simulink model "Attitude_control_RW"  (R2021b)
settings: Solver=VariableStepAuto  StartTime=0.0  StopTime=20  FixedStep=0.0001  RelTol=1e-3
values from neighbouring files (symbols this model uses):
  D = 9.4e-5*Kt    (= 4.7e-06)    [motor_parameter.m]
  J = 1.94e-4*Kt    (= 9.7e-06)    [motor_parameter.m]
  kii = (J*(-Kt^2+kpo*R)*wn^2)/(Kt*(D^2+kpo^2+J^2*wn^2-2*J*kpo*wn*zeta+2*D*(kpo-J*wn*zeta)))    (= 0.394297267374)    [motor_parameter.m]
  kpi = -(D^2*R+J^2*R*wn^2+kpo*(Kt^2-2*J*R*wn*zeta)+D*(Kt^2+R*(kpo-2*J*wn*zeta))/(Kt*(D^2+kpo^2+J^2*wn^2-2*J*kpo*wn*zeta+2*D*(kpo-J*wn*zeta))))    (= 0.0794485412984)    [motor_parameter.m]
  kpo = 10    [motor_parameter.m]
  Kt = 0.05    [motor_parameter.m]
  L = 0.001    [motor_parameter.m]
  R = 14.3    [motor_parameter.m]
  Tc = 0.053*Kt    (= 0.00265)    [motor_parameter.m]
undefined symbols (not defined in the file or in its folder): b, Is, kk, Km, Q, q_init, Rgyro, Rstr, rw_Inertia, rw_SensorToBody, Ts, unit7, w0, w_dot_init, w_init, wRW_init
libraries: simulink_extras x13, sharedtransform x12, simulink x4, slpidlib x3, aerolibutil x2, sharedTrackingLibrary x1
(part 2 of 2)

== system Attitude_control_RW/Dynamic/Subsystem ==
  qest : Inport
  Quaternions to Direction Cosine Matrix : sharedtransform/Quaternions to  Direction Cosine Matrix  aMode=aMode
      settings: SourceProductBaseCode=AE,PW,DR,MT,UV,VE
  Subsystem : Subsystem
  "DCM " : Outport  VectorParamsAs1DForOutWhenUnconnected=off
  wires:
  Quaternions to Direction Cosine Matrix/1 -> "DCM "/1
  Subsystem/1(q0,q1,q2,q3) -> Quaternions to Direction Cosine Matrix/1
  qest/1 -> Subsystem/1(q1,q2,q3,q4)

== system Attitude_control_RW/Dynamic/Subsystem1 ==
  "DCM " : Inport
  Direction Cosine Matrix to Rotation Angles : sharedtransform/Direction Cosine Matrix to Rotation Angles  rotationOrder=ZYX  aMode=aMode  action=None  tolerance=eps(2)
      settings: SourceProductBaseCode=AE,PW,DR,MT,UV,VE
  Radians to Degrees1 : simulink_extras/Transformations/Radians to Degrees
  Euler Angle : Outport  VectorParamsAs1DForOutWhenUnconnected=off
  wires:
  Radians to Degrees1/1 -> Euler Angle/1
  Direction Cosine Matrix to Rotation Angles/1 -> Radians to Degrees1/1
  "DCM "/1 -> Direction Cosine Matrix to Rotation Angles/1

== system Attitude_control_RW/Satellite Kinematic & Dynamic Model/Dynamic Model ==
  Mc+Md : Inport
  "Hrw_B " : Inport  Port=2
  Add : Sum  Inputs=-+
  Add1 : Sum
  Embedded MATLAB Function : MATLAB Function  TreatAsAtomicUnit=on
  IC : InitialCondition  Value=w_init
  IC1 : InitialCondition  Value=w_dot_init
  Inertia Matrix : Constant  Value=Is  VectorParams1D=off
  Integrator : Integrator  InitialConditionSource=external  InitialCondition=[0;0;0]
  Invert 3x3 Matrix : aerolibutil/Invert  3x3 Matrix
  Product : Product  Multiplication=Matrix(*)  RndMeth=Zero
  Product1 : Product  Multiplication=Matrix(*)  RndMeth=Zero
  Reshape : Reshape  OutputDimensionality=Column vector (2-D)
  Reshape1 : Reshape  OutputDimensionality=Column vector (2-D)
  w_initial : Constant  Value=w_init  VectorParams1D=off  SampleTime=-1
  w_IB_B : Outport  VectorParamsAs1DForOutWhenUnconnected=off
  wires:
  Inertia Matrix/1 -> Invert 3x3 Matrix/1, Product/1
  IC/1 -> Product/2, Embedded MATLAB Function/1(w)
  Mc+Md/1 -> Reshape1/1
  Invert 3x3 Matrix/1 -> Product1/1
  Integrator/1 -> w_IB_B/1, IC/1
  Product1/1 -> IC1/1
  Embedded MATLAB Function/1(y) -> Reshape/1
  w_initial/1 -> Integrator/2
  Add/1 -> Product1/2
  IC1/1 -> Integrator/1
  Reshape/1 -> Add/1
  Reshape1/1 -> Add/2
  Product/1 -> Add1/1
  Add1/1 -> Embedded MATLAB Function/2(Iw_plus_hwheel)
  "Hrw_B "/1 -> Add1/2

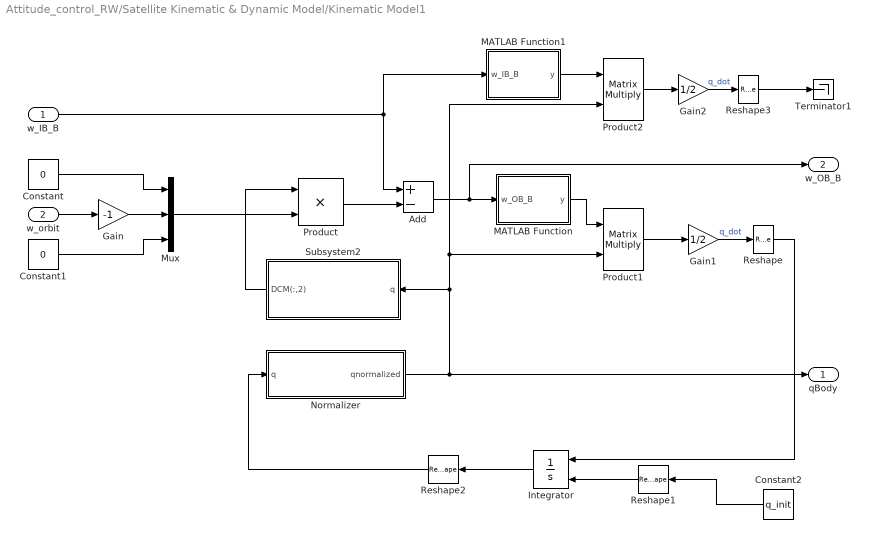
== system Attitude_control_RW/Satellite Kinematic & Dynamic Model/Kinematic Model1 ==
  w_IB_B : Inport
  w_orbit : Inport  Port=2
  Add : Sum  Inputs=+-
  Constant : Constant  Value=0
  Constant1 : Constant  Value=0
  Constant2 : Constant  Value=q_init
  Gain : Gain  Gain=-1
  Gain1 : Gain  Gain=1/2
  Gain2 : Gain  Gain=1/2
  Integrator : Integrator  InitialConditionSource=external
  MATLAB Function : MATLAB Function  TreatAsAtomicUnit=on
  MATLAB Function1 : MATLAB Function  TreatAsAtomicUnit=on
  Mux : Mux  Inputs=3
  Normalizer : MATLAB Function  TreatAsAtomicUnit=on
  Product : Product
  Product1 : Product  Multiplication=Matrix(*)
  Product2 : Product  Multiplication=Matrix(*)
  Reshape{,1..3} (4 alike) : Reshape  OutputDimensionality=Column vector (2-D)
  Subsystem2 : Subsystem
  Terminator1 : Terminator
  qBody : Outport  VectorParamsAs1DForOutWhenUnconnected=off
  w_OB_B : Outport  Port=2  VectorParamsAs1DForOutWhenUnconnected=off
  wires:
  Reshape2/1 -> Normalizer/1(q)
  Product/1 -> Add/2
  Integrator/1 -> Reshape2/1
  Normalizer/1(qnormalized) -> qBody/1, Subsystem2/1(q), Product1/2, Product2/2
  Reshape1/1 -> Integrator/2
  Add/1 -> MATLAB Function/1(w_OB_B), w_OB_B/1
  w_orbit/1 -> Gain/1
  Mux/1 -> Product/2
  Constant/1 -> Mux/1
  Constant1/1 -> Mux/3
  Product1/1 -> Gain1/1
  MATLAB Function/1(y) -> Product1/1
  Gain1/1 -> Reshape/1  "q_dot"
  w_IB_B/1 -> MATLAB Function1/1(w_IB_B), Add/1
  Product2/1 -> Gain2/1
  MATLAB Function1/1(y) -> Product2/1
  Gain2/1 -> Reshape3/1  "q_dot"
  Subsystem2/1(DCM(:,2)) -> Product/1
  Gain/1 -> Mux/2
  Reshape/1 -> Integrator/1
  Reshape3/1 -> Terminator1/1
  Constant2/1 -> Reshape1/1

== system Attitude_control_RW/Satellite Kinematic & Dynamic Model/Subsystem ==
  qest : Inport
  Quaternions to Direction Cosine Matrix : sharedtransform/Quaternions to  Direction Cosine Matrix  aMode=aMode
      settings: SourceProductBaseCode=AE
  Subsystem : Subsystem
  "DCM " : Outport  VectorParamsAs1DForOutWhenUnconnected=off
  wires:
  Quaternions to Direction Cosine Matrix/1 -> "DCM "/1
  Subsystem/1(q0,q1,q2,q3) -> Quaternions to Direction Cosine Matrix/1
  qest/1 -> Subsystem/1(q1,q2,q3,q4)

== system Attitude_control_RW/Satellite Kinematic & Dynamic Model/Subsystem1 ==
  "DCM " : Inport
  Direction Cosine Matrix to Rotation Angles : sharedtransform/Direction Cosine Matrix to Rotation Angles  rotationOrder=ZYX  aMode=aMode  action=None  tolerance=eps(2)
      settings: SourceProductBaseCode=AE
  Radians to Degrees1 : simulink_extras/Transformations/Radians to Degrees
  Euler Angle : Outport  VectorParamsAs1DForOutWhenUnconnected=off
  wires:
  Radians to Degrees1/1 -> Euler Angle/1
  Direction Cosine Matrix to Rotation Angles/1 -> Radians to Degrees1/1
  "DCM "/1 -> Direction Cosine Matrix to Rotation Angles/1

== system Attitude_control_RW/Sensor Measurement Model (GYRO + STR)/GYRO Sensor Model ==
  w_Body : Inport
  Gyroscope Model : Subsystem
  Zero-Order Hold2 : ZeroOrderHold  SampleTime=Ts
  w_Body_meas : Outport  VectorParamsAs1DForOutWhenUnconnected=off
  wires:
  w_Body/1 -> Gyroscope Model/1(w_Body)
  Gyroscope Model/1(Gyro1_wmeas) -> Zero-Order Hold2/1
  Zero-Order Hold2/1 -> w_Body_meas/1

== system Attitude_control_RW/Sensor Measurement Model (GYRO + STR)/Normalization Model ==
  u : Inport
  Divide : Product  Inputs=*/
  MATLAB Function : MATLAB Function  TreatAsAtomicUnit=on
  Math Function2 : Math  Operator=square  SignedPower=on  SaturateOnIntegerOverflow=on
  Sum of Elements : Sum  Inputs=+
  Normalized_u : Outport  VectorParamsAs1DForOutWhenUnconnected=off
  wires:
  Divide/1 -> Normalized_u/1
  MATLAB Function/1(y) -> Divide/2
  Sum of Elements/1 -> MATLAB Function/1(u)
  u/1 -> Divide/1, Math Function2/1
  Math Function2/1 -> Sum of Elements/1

== system Attitude_control_RW/Sensor Measurement Model (GYRO + STR)/Star Tracker Model ==
  q_Body : Inport
  Scope : Scope
  StarTracker 1 Error Model3 : Subsystem  TreatAsAtomicUnit=on
  Zero-Order Hold2 : ZeroOrderHold  SampleTime=0.1
  q_Body_meas : Outport  VectorParamsAs1DForOutWhenUnconnected=off
  wires:
  Zero-Order Hold2/1 -> Scope/1, q_Body_meas/1
  q_Body/1 -> StarTracker 1 Error Model3/1("q_Body ")
  StarTracker 1 Error Model3/1("q_body_meas ") -> Zero-Order Hold2/1

== system Attitude_control_RW/Subsystem/Subsystem1 ==
  q0,q1,q2,q3 : Inport
  Demux1 : Demux
  Mux1 : Mux
  q1,q2,q3,q4 : Outport  VectorParamsAs1DForOutWhenUnconnected=off
  wires:
  q0,q1,q2,q3/1 -> Demux1/1
  Mux1/1 -> q1,q2,q3,q4/1
  Demux1/1 -> Mux1/4
  Demux1/2 -> Mux1/1
  Demux1/3 -> Mux1/2
  Demux1/4 -> Mux1/3

== system Attitude_control_RW/Subsystem1/Subsystem1 ==
  q0,q1,q2,q3 : Inport
  Demux1 : Demux
  Mux1 : Mux
  q1,q2,q3,q4 : Outport  VectorParamsAs1DForOutWhenUnconnected=off
  wires:
  q0,q1,q2,q3/1 -> Demux1/1
  Mux1/1 -> q1,q2,q3,q4/1
  Demux1/1 -> Mux1/4
  Demux1/2 -> Mux1/1
  Demux1/3 -> Mux1/2
  Demux1/4 -> Mux1/3

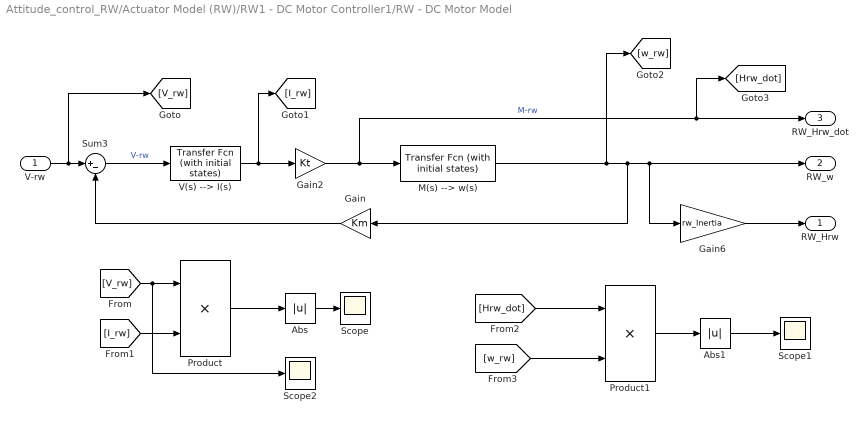
== system Attitude_control_RW/Actuator Model (RW)/RW1 - DC Motor Controller1/RW - DC Motor Model ==
  V-rw : Inport
  Abs : Abs
  Abs1 : Abs
  Gain : Gain  Gain=Km
  Gain2 : Gain  Gain=Kt
  Gain6 : Gain  Gain=rw_Inertia
  M(s) --> w(s) : simulink_extras/Additional Linear/Transfer Fcn (with initial states)  N=[1]  D=[5e-4 b]  X0=0
  Product : Product
  Product1 : Product
  Scope : Scope
  Scope1 : Scope
  Scope2 : Scope
  Sum3 : Sum  Inputs=|+-
  V(s) --> I(s) : simulink_extras/Additional Linear/Transfer Fcn (with initial states)  N=1  D=[R]  X0=0
  RW_Hrw : Outport  VectorParamsAs1DForOutWhenUnconnected=off
  RW_w : Outport  Port=2  VectorParamsAs1DForOutWhenUnconnected=off
  RW_Hrw_dot : Outport  Port=3  VectorParamsAs1DForOutWhenUnconnected=off
  wires:
  V-rw/1 -> [V_rw], Sum3/1
  Gain2/1 -> M(s) --> w(s)/1, [Hrw_dot], RW_Hrw_dot/1  "M-rw"
  Gain6/1 -> RW_Hrw/1
  Gain/1 -> Sum3/2
  Sum3/1 -> V(s) --> I(s)/1  "V-rw"
  V(s) --> I(s)/1 -> [I_rw], Gain2/1
  M(s) --> w(s)/1 -> RW_w/1, Gain6/1, Gain/1, [w_rw]
  [V_rw] -> Scope2/1, Product/1
  [I_rw] -> Product/2
  Product/1 -> Abs/1
  Abs/1 -> Scope/1
  [Hrw_dot] -> Product1/1
  [w_rw] -> Product1/2
  Product1/1 -> Abs1/1
  Abs1/1 -> Scope1/1

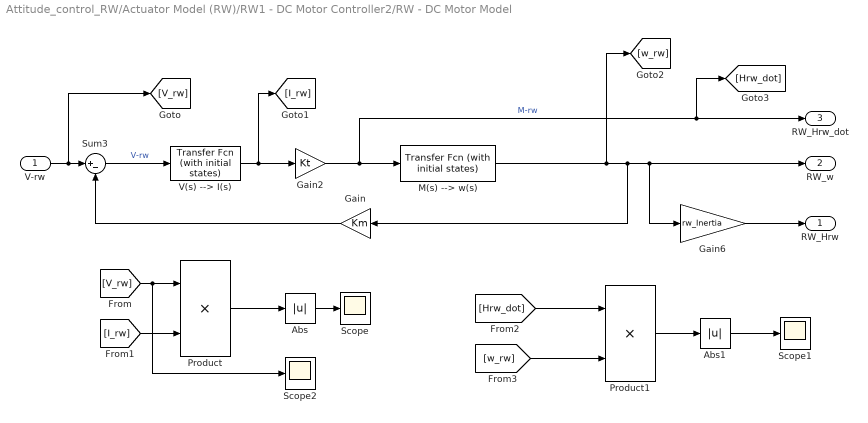
== system Attitude_control_RW/Actuator Model (RW)/RW1 - DC Motor Controller2/RW - DC Motor Model ==
  V-rw : Inport
  Abs : Abs
  Abs1 : Abs
  Gain : Gain  Gain=Km
  Gain2 : Gain  Gain=Kt
  Gain6 : Gain  Gain=rw_Inertia
  M(s) --> w(s) : simulink_extras/Additional Linear/Transfer Fcn (with initial states)  N=[1]  D=[5e-4 b]  X0=0
  Product : Product
  Product1 : Product
  Scope : Scope
  Scope1 : Scope
  Scope2 : Scope
  Sum3 : Sum  Inputs=|+-
  V(s) --> I(s) : simulink_extras/Additional Linear/Transfer Fcn (with initial states)  N=1  D=[R]  X0=0
  RW_Hrw : Outport  VectorParamsAs1DForOutWhenUnconnected=off
  RW_w : Outport  Port=2  VectorParamsAs1DForOutWhenUnconnected=off
  RW_Hrw_dot : Outport  Port=3  VectorParamsAs1DForOutWhenUnconnected=off
  wires:
  V-rw/1 -> [V_rw], Sum3/1
  Gain2/1 -> M(s) --> w(s)/1, [Hrw_dot], RW_Hrw_dot/1  "M-rw"
  Gain6/1 -> RW_Hrw/1
  Gain/1 -> Sum3/2
  Sum3/1 -> V(s) --> I(s)/1  "V-rw"
  V(s) --> I(s)/1 -> [I_rw], Gain2/1
  M(s) --> w(s)/1 -> RW_w/1, Gain6/1, Gain/1, [w_rw]
  [V_rw] -> Scope2/1, Product/1
  [I_rw] -> Product/2
  Product/1 -> Abs/1
  Abs/1 -> Scope/1
  [Hrw_dot] -> Product1/1
  [w_rw] -> Product1/2
  Product1/1 -> Abs1/1
  Abs1/1 -> Scope1/1

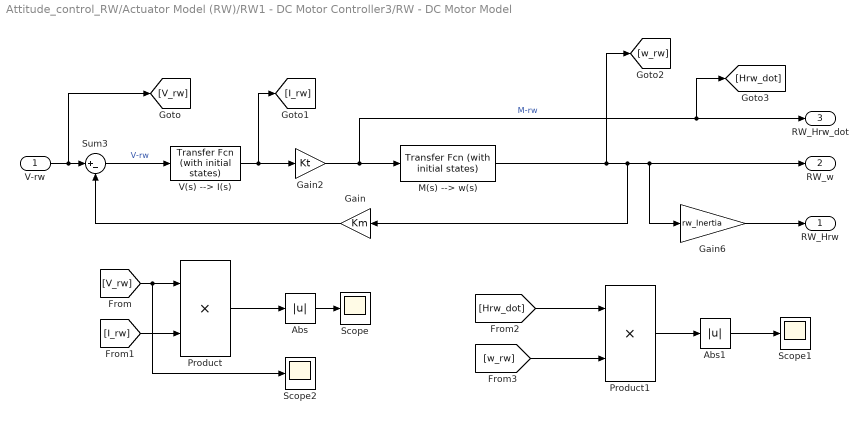
== system Attitude_control_RW/Actuator Model (RW)/RW1 - DC Motor Controller3/RW - DC Motor Model ==
  V-rw : Inport
  Abs : Abs
  Abs1 : Abs
  Gain : Gain  Gain=Km
  Gain2 : Gain  Gain=Kt
  Gain6 : Gain  Gain=rw_Inertia
  M(s) --> w(s) : simulink_extras/Additional Linear/Transfer Fcn (with initial states)  N=[1]  D=[5e-4 b]  X0=0
  Product : Product
  Product1 : Product
  Scope : Scope
  Scope1 : Scope
  Scope2 : Scope
  Sum3 : Sum  Inputs=|+-
  V(s) --> I(s) : simulink_extras/Additional Linear/Transfer Fcn (with initial states)  N=1  D=[R]  X0=0
  RW_Hrw : Outport  VectorParamsAs1DForOutWhenUnconnected=off
  RW_w : Outport  Port=2  VectorParamsAs1DForOutWhenUnconnected=off
  RW_Hrw_dot : Outport  Port=3  VectorParamsAs1DForOutWhenUnconnected=off
  wires:
  V-rw/1 -> [V_rw], Sum3/1
  Gain2/1 -> M(s) --> w(s)/1, [Hrw_dot], RW_Hrw_dot/1  "M-rw"
  Gain6/1 -> RW_Hrw/1
  Gain/1 -> Sum3/2
  Sum3/1 -> V(s) --> I(s)/1  "V-rw"
  V(s) --> I(s)/1 -> [I_rw], Gain2/1
  M(s) --> w(s)/1 -> RW_w/1, Gain6/1, Gain/1, [w_rw]
  [V_rw] -> Scope2/1, Product/1
  [I_rw] -> Product/2
  Product/1 -> Abs/1
  Abs/1 -> Scope/1
  [Hrw_dot] -> Product1/1
  [w_rw] -> Product1/2
  Product1/1 -> Abs1/1
  Abs1/1 -> Scope1/1

== system Attitude_control_RW/Actuator Model (RW)/RW1 - DC Motor Controller5/RW - DC Motor Model ==
  V-rw : Inport
  Abs : Abs
  Abs1 : Abs
  Gain : Gain  Gain=Km
  Gain2 : Gain  Gain=Kt
  Gain6 : Gain  Gain=rw_Inertia
  M(s) --> w(s) : simulink_extras/Additional Linear/Transfer Fcn (with initial states)  N=[1]  D=[5e-4 b]  X0=0
  Product : Product
  Product1 : Product
  Scope : Scope
  Scope1 : Scope
  Scope2 : Scope
  Sum3 : Sum  Inputs=|+-
  V(s) --> I(s) : simulink_extras/Additional Linear/Transfer Fcn (with initial states)  N=1  D=[R]  X0=0
  RW_Hrw : Outport  VectorParamsAs1DForOutWhenUnconnected=off
  RW_w : Outport  Port=2  VectorParamsAs1DForOutWhenUnconnected=off
  RW_Hrw_dot : Outport  Port=3  VectorParamsAs1DForOutWhenUnconnected=off
  wires:
  V-rw/1 -> [V_rw], Sum3/1
  Gain2/1 -> M(s) --> w(s)/1, [Hrw_dot], RW_Hrw_dot/1  "M-rw"
  Gain6/1 -> RW_Hrw/1
  Gain/1 -> Sum3/2
  Sum3/1 -> V(s) --> I(s)/1  "V-rw"
  V(s) --> I(s)/1 -> [I_rw], Gain2/1
  M(s) --> w(s)/1 -> RW_w/1, Gain6/1, Gain/1, [w_rw]
  [V_rw] -> Scope2/1, Product/1
  [I_rw] -> Product/2
  Product/1 -> Abs/1
  Abs/1 -> Scope/1
  [Hrw_dot] -> Product1/1
  [w_rw] -> Product1/2
  Product1/1 -> Abs1/1
  Abs1/1 -> Scope1/1

== system Attitude_control_RW/Controller/Subsystem/Subsystem1 ==
  q0,q1,q2,q3 : Inport
  Demux1 : Demux
  Mux1 : Mux
  q1,q2,q3,q4 : Outport  VectorParamsAs1DForOutWhenUnconnected=off
  wires:
  q0,q1,q2,q3/1 -> Demux1/1
  Mux1/1 -> q1,q2,q3,q4/1
  Demux1/1 -> Mux1/4
  Demux1/2 -> Mux1/1
  Demux1/3 -> Mux1/2
  Demux1/4 -> Mux1/3

== system Attitude_control_RW/Dynamic/Kinematic Model1/Subsystem2 ==
  q : Inport
  MATLAB Function : MATLAB Function  TreatAsAtomicUnit=on
  Quaternions to Direction Cosine Matrix : sharedtransform/Quaternions to  Direction Cosine Matrix  aMode=aMode
      settings: SourceProductBaseCode=AE,PW,DR,MT,UV,VE
  Reshape2 : Reshape  OutputDimensionality=Column vector (2-D)
  Subsystem : Subsystem
  DCM(:,2) : Outport  VectorParamsAs1DForOutWhenUnconnected=off
  wires:
  Subsystem/1(q0,q1,q2,q3) -> Quaternions to Direction Cosine Matrix/1
  q/1 -> Subsystem/1(q1,q2,q3,q4)
  Quaternions to Direction Cosine Matrix/1 -> MATLAB Function/1(DCM)
  MATLAB Function/1(DCM_2) -> Reshape2/1
  Reshape2/1 -> DCM(:,2)/1

== system Attitude_control_RW/Dynamic/Subsystem/Subsystem ==
  q1,q2,q3,q4 : Inport
  Demux1 : Demux
  Mux1 : Mux
  q0,q1,q2,q3 : Outport  VectorParamsAs1DForOutWhenUnconnected=off
  wires:
  Demux1/2 -> Mux1/3
  q1,q2,q3,q4/1 -> Demux1/1
  Mux1/1 -> q0,q1,q2,q3/1
  Demux1/4 -> Mux1/1
  Demux1/1 -> Mux1/2
  Demux1/3 -> Mux1/4

== system Attitude_control_RW/Satellite Kinematic & Dynamic Model/Kinematic Model1/Subsystem2 ==
  q : Inport
  MATLAB Function : MATLAB Function  TreatAsAtomicUnit=on
  Quaternions to Direction Cosine Matrix : sharedtransform/Quaternions to  Direction Cosine Matrix  aMode=aMode
      settings: SourceProductBaseCode=AE
  Reshape2 : Reshape  OutputDimensionality=Column vector (2-D)
  Subsystem : Subsystem
  DCM(:,2) : Outport  VectorParamsAs1DForOutWhenUnconnected=off
  wires:
  Subsystem/1(q0,q1,q2,q3) -> Quaternions to Direction Cosine Matrix/1
  q/1 -> Subsystem/1(q1,q2,q3,q4)
  Quaternions to Direction Cosine Matrix/1 -> MATLAB Function/1(DCM)
  MATLAB Function/1(DCM_2) -> Reshape2/1
  Reshape2/1 -> DCM(:,2)/1

== system Attitude_control_RW/Satellite Kinematic & Dynamic Model/Subsystem/Subsystem ==
  q1,q2,q3,q4 : Inport
  Demux1 : Demux
  Mux1 : Mux
  q0,q1,q2,q3 : Outport  VectorParamsAs1DForOutWhenUnconnected=off
  wires:
  Demux1/2 -> Mux1/3
  q1,q2,q3,q4/1 -> Demux1/1
  Mux1/1 -> q0,q1,q2,q3/1
  Demux1/4 -> Mux1/1
  Demux1/1 -> Mux1/2
  Demux1/3 -> Mux1/4

== system Attitude_control_RW/Sensor Measurement Model (GYRO + STR)/GYRO Sensor Model/Gyroscope Model ==
  w_Body : Inport
  Add : Sum
  Band-Limited White Noise : simulink/Sources/Band-Limited White Noise  Cov=Rgyro*Ts  Ts=Ts  seed=[23341]
  Saturation1 : Saturate  UpperLimit=abs(1000)  LowerLimit=-abs(1000)
  Gyro1_wmeas : Outport  VectorParamsAs1DForOutWhenUnconnected=off
  wires:
  Add/1 -> Saturation1/1
  Saturation1/1 -> Gyro1_wmeas/1
  w_Body/1 -> Add/1
  Band-Limited White Noise/1 -> Add/2

== system Attitude_control_RW/Sensor Measurement Model (GYRO + STR)/Star Tracker Model/StarTracker 1 Error Model3 ==
  "q_Body " : Inport
  Add : Sum
  Band-Limited White Noise : simulink/Sources/Band-Limited White Noise  Cov=Rstr*Ts  Ts=Ts  seed=[12345]
  "q_body_meas " : Outport  VectorParamsAs1DForOutWhenUnconnected=off
  wires:
  Band-Limited White Noise/1 -> Add/2
  "q_Body "/1 -> Add/1
  Add/1 -> "q_body_meas "/1

== system Attitude_control_RW/Dynamic/Kinematic Model1/Subsystem2/Subsystem ==
  q1,q2,q3,q4 : Inport
  Demux1 : Demux
  Mux1 : Mux
  q0,q1,q2,q3 : Outport  VectorParamsAs1DForOutWhenUnconnected=off
  wires:
  Demux1/2 -> Mux1/3
  q1,q2,q3,q4/1 -> Demux1/1
  Mux1/1 -> q0,q1,q2,q3/1
  Demux1/4 -> Mux1/1
  Demux1/1 -> Mux1/2
  Demux1/3 -> Mux1/4

== system Attitude_control_RW/Satellite Kinematic & Dynamic Model/Kinematic Model1/Subsystem2/Subsystem ==
  q1,q2,q3,q4 : Inport
  Demux1 : Demux
  Mux1 : Mux
  q0,q1,q2,q3 : Outport  VectorParamsAs1DForOutWhenUnconnected=off
  wires:
  Demux1/2 -> Mux1/3
  q1,q2,q3,q4/1 -> Demux1/1
  Mux1/1 -> q0,q1,q2,q3/1
  Demux1/4 -> Mux1/1
  Demux1/1 -> Mux1/2
  Demux1/3 -> Mux1/4

== matlab function Attitude_control_RW/Satellite Kinematic & Dynamic Model/Kinematic Model1/Normalizer ==
  data: qnormalized output; q input
function qnormalized = fcn(q)

%Normalizes the quaternion

qnormalized = q;
qs = q(4);
qv = [q(1); q(2); q(3)];

qnormalized(4)= qs /norm(q);
qnormalized(1)= qv(1)/norm(q);
qnormalized(2)= qv(2)/norm(q);
qnormalized(3)= qv(3)/norm(q);

== matlab function Attitude_control_RW/Dynamic/Kinematic Model1/MATLAB Function1 ==
  data: w_IB_B input; y output
function y = skew_wIB_B(w_IB_B)


y = [0, w_IB_B(3,1), -w_IB_B(2,1), w_IB_B(1,1);...
    -w_IB_B(3,1), 0, w_IB_B(1,1), w_IB_B(2,1);...
     w_IB_B(2,1), -w_IB_B(1,1), 0, w_IB_B(3,1);...
    -w_IB_B(1,1), -w_IB_B(2,1), -w_IB_B(3,1), 0];
end

== matlab function Attitude_control_RW/Actuator Model (RW)/Reaction Wheel Model ==
  data: rw_SensorToBody input; Hrw_dot_des output; inv_rwSensorToBody input; Mc input; w_IB_B input; wRw input
function Hrw_dot_des = rwModel(rw_SensorToBody,inv_rwSensorToBody,Mc,w_IB_B,wRw)
% The desired torque is calculated for each reaction wheel 

% The required momentum input
% wRw               (4x1) matrix
% rwInertia_matrix  (4x4) matrix
% rw_SensorToBody   (3x4) matrix
rwInertia = 5e-4; % RW moment of inertia (kg-m2)
rwInertia_matrix = eye(4,4)* rwInertia;
Hrw = rwInertia_matrix * wRw; 

% Hrw_B     (3x1) matrix
% Hrw_B_dot (3x1) matrix
% From Actuator Frame to Satellite Body Frame
Hrw_B = rw_SensorToBody * Hrw ;

% Desired reaction wheel torque in Body Frame
Hrw_B_dot = Mc + cross(w_IB_B,Hrw_B) ;

% Desired reaction wheel torque in Actuator Frame
Hrw_dot_des = inv_rwSensorToBody * Hrw_B_dot ; 

end

== matlab function Attitude_control_RW/Actuator Model (RW)/RW1 - DC Motor Controller5/MATLAB Function1 ==
  data: y output
function y = fcn()
sigma = 2;
y = sigma*randn;

== matlab function Attitude_control_RW/MATLAB Function ==
  data: qref input; qerr_xyz output; qest input
function qerr_xyz  = quaternionError(qref, qest)

qerr = [qest(4)  qest(3) -qest(2) qest(1);...
       -qest(3)  qest(4)  qest(1) qest(2);...
        qest(2) -qest(1)  qest(4) qest(3);...
       -qest(1) -qest(2) -qest(3) qest(4)]*[-qref(1);-qref(2);-qref(3);qref(4)]; % Verify

qerr_xyz = [qerr(1,1); qerr(2,1); qerr(3,1)];     
% qerr_x = qerr(1,1);
% qerr_y = qerr(2,1);
% qerr_z = qerr(3,1);
qerr_4 = qerr(4,1);
qerr_xyz*qerr_4;

end
% % 
% function qerr_xyz  = quaternionError(qref, qest)
% 
% qerr = [qref(4)  -qref(3) qref(2) qref(1);...
%         qref(3)  qref(4)  -qref(1) qref(2);...
%         -qref(2) qref(1)  qref(4) qref(3);...
%        -qref(1) -qref(2) -qref(3) qref(4)]*[-qest(1);-qest(2);-qest(3);qest(4)];
% 
% qerr_xyz = [qerr(1,1); qerr(2,1); qerr(3,1)];     
% % qerr_x = qerr(1,1);
% % qerr_y = qerr(2,1);
% % qerr_z = qerr(3,1);
% 
% end

== matlab function Attitude_control_RW/Sensor Measurement Model (GYRO + STR)/Normalization Model/MATLAB Function ==
  data: u input; y output
function y = Sqrt(u)
%#codegen

y = sqrt(u);

== matlab function Attitude_control_RW/Actuator Model (RW)/RW1 - DC Motor Controller5/MATLAB Function ==
  data: y output
function y = fcn()
sigma = 0.1;
y = sigma*randn;

== matlab function Attitude_control_RW/Controller/MATLAB Function ==
  data: qref input; qerr_xyz output; qest input
function qerr_xyz  = quaternionError(qref, qest)

qerr = [qest(4)  qest(3) -qest(2) qest(1);...
       -qest(3)  qest(4)  qest(1) qest(2);...
        qest(2) -qest(1)  qest(4) qest(3);...
       -qest(1) -qest(2) -qest(3) qest(4)]*[-qref(1);-qref(2);-qref(3);qref(4)]; % Verify

qerr_xyz = [qerr(1,1); qerr(2,1); qerr(3,1)];     
% qerr_x = qerr(1,1);
% qerr_y = qerr(2,1);
% qerr_z = qerr(3,1);
qerr_4 = qerr(4,1);
qerr_xyz*qerr_4;

end
% % 
% function qerr_xyz  = quaternionError(qref, qest)
% 
% qerr = [qref(4)  -qref(3) qref(2) qref(1);...
%         qref(3)  qref(4)  -qref(1) qref(2);...
%         -qref(2) qref(1)  qref(4) qref(3);...
%        -qref(1) -qref(2) -qref(3) qref(4)]*[-qest(1);-qest(2);-qest(3);qest(4)];
% 
% qerr_xyz = [qerr(1,1); qerr(2,1); qerr(3,1)];     
% % qerr_x = qerr(1,1);
% % qerr_y = qerr(2,1);
% % qerr_z = qerr(3,1);
% 
% end

== matlab function Attitude_control_RW/Dynamic/Dynamic Model/Embedded MATLAB Function ==
  data: w input; y output; Iw_plus_hwheel input
function y = crossproduct(w, Iw_plus_hwheel)


y = cross(w,Iw_plus_hwheel);

== matlab function Attitude_control_RW/MATLAB Function1 ==
  data: w_IB_B input; w_OB_B output; q_Body input; w_O input
function w_OB_B = fcn(w_IB_B,q_Body,w_O)


w_OB_B = [w_IB_B(1)+2*(q_Body(1)*q_Body(2)+q_Body(3)*q_Body(4))*w_O;
          w_IB_B(2)+w_O*(q_Body(4)^2-q_Body(1)^2+q_Body(2)^2-q_Body(3)^2);
          w_IB_B(3)+2*(q_Body(2)*q_Body(3)-q_Body(1)*q_Body(4))*w_O];

== matlab function Attitude_control_RW/MATLAB Function2 ==
  data: qref input; qerr_xyz output; qest input
function qerr_xyz  = quaternionError(qref, qest)

qerr = [qest(4)  qest(3) -qest(2) qest(1);...
       -qest(3)  qest(4)  qest(1) qest(2);...
        qest(2) -qest(1)  qest(4) qest(3);...
       -qest(1) -qest(2) -qest(3) qest(4)]*[-qref(1);-qref(2);-qref(3);qref(4)];

qerr_xyz = [qerr(1,1); qerr(2,1); qerr(3,1)];     
% qerr_x = qerr(1,1);
% qerr_y = qerr(2,1);
% qerr_z = qerr(3,1);

end
% % 
% function qerr_xyz  = quaternionError(qref, qest)
% 
% qerr = [qref(4)  -qref(3) qref(2) qref(1);...
%         qref(3)  qref(4)  -qref(1) qref(2);...
%         -qref(2) qref(1)  qref(4) qref(3);...
%        -qref(1) -qref(2) -qref(3) qref(4)]*[-qest(1);-qest(2);-qest(3);qest(4)];
% 
% qerr_xyz = [qerr(1,1); qerr(2,1); qerr(3,1)];     
% % qerr_x = qerr(1,1);
% % qerr_y = qerr(2,1);
% % qerr_z = qerr(3,1);
% 
% end

== matlab function Attitude_control_RW/Dynamic/Kinematic Model1/Subsystem2/MATLAB Function ==
  data: DCM input; DCM_2 output
function DCM_2 = fcn(DCM)
DCM_2 = DCM(:,2);
end

== matlab function Attitude_control_RW/Satellite Kinematic & Dynamic Model/Dynamic Model/Embedded MATLAB Function ==
  data: w input; y output; Iw_plus_hwheel input
function y = crossproduct(w,Iw_plus_hwheel)
% This block supports the Embedded MATLAB subset.
% See the help menu for details. 

%Just used to calculate the cross-product of two inputs
y = cross(w,Iw_plus_hwheel);

== matlab function Attitude_control_RW/Satellite Kinematic & Dynamic Model/Kinematic Model1/MATLAB Function ==
  data: w_OB_B input; y output
function y = skew_wOB_B(w_OB_B)


y = [0, w_OB_B(3,1), -w_OB_B(2,1), w_OB_B(1,1);...
    -w_OB_B(3,1), 0, w_OB_B(1,1), w_OB_B(2,1);...
     w_OB_B(2,1), -w_OB_B(1,1), 0, w_OB_B(3,1);...
    -w_OB_B(1,1), -w_OB_B(2,1), -w_OB_B(3,1), 0];
end

== matlab function Attitude_control_RW/Satellite Kinematic & Dynamic Model/Kinematic Model1/MATLAB Function1 ==
  data: w_IB_B input; y output
function y = skew_wIB_B(w_IB_B)


y = [0, w_IB_B(3,1), -w_IB_B(2,1), w_IB_B(1,1);...
    -w_IB_B(3,1), 0, w_IB_B(1,1), w_IB_B(2,1);...
     w_IB_B(2,1), -w_IB_B(1,1), 0, w_IB_B(3,1);...
    -w_IB_B(1,1), -w_IB_B(2,1), -w_IB_B(3,1), 0];
end

== matlab function Attitude_control_RW/Satellite Kinematic & Dynamic Model/Kinematic Model1/Subsystem2/MATLAB Function ==
  data: DCM input; DCM_2 output
function DCM_2 = fcn(DCM)
DCM_2 = DCM(:,2);
end

== matlab function Attitude_control_RW/Dynamic/Kinematic Model1/MATLAB Function ==
  data: w_OB_B input; y output
function y = skew_wOB_B(w_OB_B)


y = [0, w_OB_B(3,1), -w_OB_B(2,1), w_OB_B(1,1);...
    -w_OB_B(3,1), 0, w_OB_B(1,1), w_OB_B(2,1);...
     w_OB_B(2,1), -w_OB_B(1,1), 0, w_OB_B(3,1);...
    -w_OB_B(1,1), -w_OB_B(2,1), -w_OB_B(3,1), 0];
end
